simulink model "ce1_1_sim"  (R2016b)
settings: Solver=VariableStepAuto  StartTime=0.0  StopTime=10.0  RelTol=1e-3  EnableMultiTasking=on
values from neighbouring files (symbols this model uses):
  Te = 0.2    [ce1_1.m]    (also in ce1_3.m; ce1_4.m; ce2_1.m; ce2_2.m)
settings Model: Creator=user  LastModifiedBy=Camilla
settings OptimizationCC: LifeSpan=inf
settings DebuggingCC: SFUnexpectedBacktrackingDiag=warning  SFNoUnconditionalDefaultTransitionDiag=warning  SFExecutionAtInitializationDiag=none
settings GRTTargetCC: TargetLangStandard=C89/C90 (ANSI)  GeneratePreprocessorConditionals=Disable all
settings ConfigComp: CovMetricSettings=dw  CovHtmlReporting=on  CovSaveCumulativeToWorkspaceVar=on  CovSaveSingleToWorkspaceVar=on  CovExternalEMLEnable=off

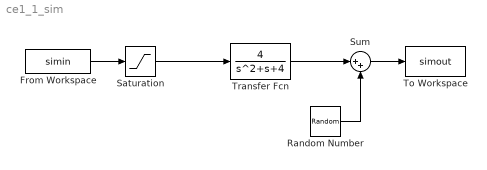
== system ce1_1_sim ==
  From Workspace : FromWorkspace  VariableName=simin  SampleTime=Te
  Random Number : RandomNumber  Variance=0.1  SampleTime=Te
  Saturation : Saturate
  Sum : Sum  Inputs=|++
  To Workspace : ToWorkspace  VariableName=simout  SaveFormat=Timeseries  SampleTime=Te
  Transfer Fcn : TransferFcn  Numerator=[4]  Denominator=[1 1 4]
  wires:
  Transfer Fcn/1 -> Sum/1
  Saturation/1 -> Transfer Fcn/1
  From Workspace/1 -> Saturation/1
  Sum/1 -> To Workspace/1
  Random Number/1 -> Sum/2
